simulink model "slexSysIdentMATLABSystemExample"  (R2017b)
settings: Solver=FixedStepDiscrete  StartTime=0.0  StopTime=1000  FixedStep=1  RelTol=1e-3
PreLoadFcn:
  | b = [ -0.0012   -0.0014    0.0020    0.0029   -0.0044   -0.0064    0.0090    0.0125 -0.0169   -0.0227    0.0305    0.0412   -0.0573   -0.0850    0.1472    0.4501 0.4501    0.1472   -0.0850   -0.0573    0.0412    0.0305   -0.0227   -0.0169 0.0125    0.0090   -0.0064   -0.0044    0.0029    0.0020   -0.0014   -0.0012];
  | N = 1;
InitFcn:
  | a = [zeros(1, N), b]; % Co-efficients of combined System (Unknown + Delay)
CloseFcn:
  | clear a b N
Description:
  | System Identification for an FIR System Using MATLAB System Blocks
  | 
  | This example shows how to use the MATLAB System block to implement
  | Simulink(R) blocks using a System object(TM). It highlights two MATLAB System blocks.
  | Access the MATLAB source code for each System object by clicking the "Source Code"
  | hyperlink from the block dialog.
  | 
  | * The Delay block uses a System object that has direct feedthrough
  | set to false. This implies that the System object does not directly use the input to
  | compute the output. Therefore, the Delay block could be safely used in a feedback system
  | without introducing an algebraic loop.
  | 
  | * The LMS Adaptive Filter block estimates the coefficients of an unknown system (formed
  | by the Unknown System and Delay blocks). Its inputs are the desired signal and
  | the actual signal. Its outputs are the estimated signal and the vector norm of the
  | error in the estimated coefficients.
  | 
  | * The Scope displays the error in the estimated signal and the vector norm
  | of the error in the estimated coefficients.
settings Model: ExtModeAutoUpdateStatusClock=off  Creator=The MathWorks, Inc.  LastModifiedBy=prave
settings DataIOCC: SaveFormat=Structure  SaveState=on
settings OptimizationCC: ExpressionDepthLimit=2147483647  InitFltsAndDblsToZero=on  LifeSpan=1
settings DebuggingCC: SaveWithParameterizedLinksMsg=none  UnderspecifiedInitializationDetection=Classic  MergeDetectMultiDrivingBlocksExec=none  SignalResolutionControl=TryResolveAllWithWarning  SolverPrmCheckMsg=warning  MultiTaskDSMMsg=warning  MultiTaskCondExecSysMsg=none  FcnCallInpInsideContextMsg=warning  AllowSymbolicDim=off  StateNameClashWarn=warning  SFUnexpectedBacktrackingDiag=warning  SFNoUnconditionalDefaultTransitionDiag=warning  SFExecutionAtInitializationDiag=none
settings HardwareCC: ProdBitPerPointer=32  ProdBitPerSizeT=32  ProdBitPerPtrDiffT=32  ProdLargestAtomicFloat=None  ProdIntDivRoundTo=Undefined  ProdEndianess=Unspecified  ProdWordSize=32  ProdHWDeviceType=32-bit Generic
settings ModelReferenceCC: PropagateSignalLabelsOutOfModel=off
settings SFSimCC: MATLABDynamicMemAlloc=off
settings RTWCC: SystemTargetFile=ert.tlc  TemplateMakefile=ert_default_tmf
settings CodeAppCC: IgnoreCustomStorageClasses=off  CustomSymbolStrType=$N$R$M  StateflowObjectComments=on  InternalIdentifier=Classic
settings ERTTargetCC: MultiwordLength=2048  GenerateSampleERTMain=on  ERTCustomFileTemplate=example_file_process.tlc  ConvertIfToSwitch=off  SuppressUnreachableDefaultCases=off
settings ConfigComp: CovMetricSettings=dw  CovHtmlReporting=on  CovSaveCumulativeToWorkspaceVar=on  CovSaveSingleToWorkspaceVar=on  CovExternalEMLEnable=off  CovSFcnEnable=off

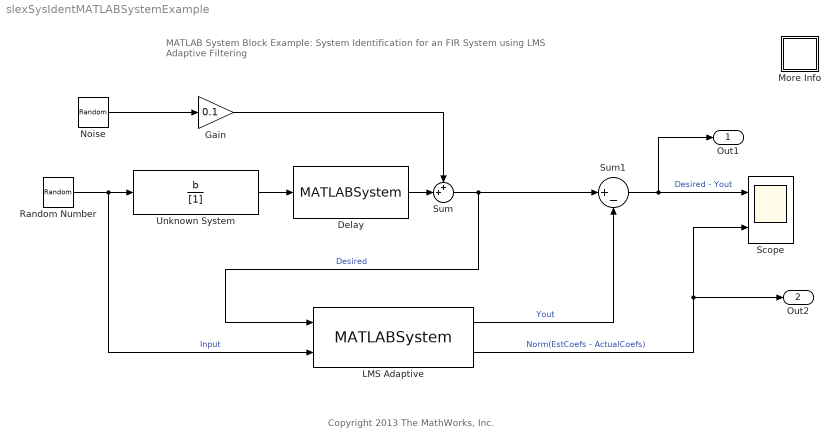
== system slexSysIdentMATLABSystemExample ==
  note: MATLAB System Block Example:
      | System Identification for an FIR System using LMS Adaptive Filtering
  note: Copyright 2013 The MathWorks, Inc.
  Delay : MATLABSystem  System=slexSysIdentMATLABSystemIntegerDelaySysObj  InitialOutput=0  NumberOfDelays=N  SimulateUsing=Code generation
      mask Type: slexSysIdentMATLABSystemIntegerDelaySysObj
      mask Display:
      | disp(['Integer' char(10) 'Delay']);
      | port_label('input',1,'inputs');
      | port_label('output',1,'outputs');
  Gain : Gain  Gain=0.1
  LMS Adaptive : MATLABSystem  System=slexSysIdentMATLABSystemLMSAdaptSysObj  Mu=0.005  SimulateUsing=Code generation  TrueCoefficients=a  NumCoefficients=numel(a)
      mask Type: slexSysIdentMATLABSystemLMSAdaptSysObj
      mask Display:
      | disp(['LMS Adaptive' char(10) 'Filter']);
      | port_label('input',1,'Desired');
      | port_label('input',2,'Actual');
      | port_label('output',1,'Output');
      | port_label('output',2,'EstError');
  More Info : Subsystem
      settings: OpenFcn=showdemo(bdroot(gcb))
      mask Display: disp('?')
  Noise : RandomNumber  Seed=3  SampleTime=1
  Random Number : RandomNumber  SampleTime=1
  Scope : Scope  NumInputPorts=2
  Sum : Sum  Inputs=++|
  Sum1 : Sum  Inputs=|+-
  Unknown System : DiscreteFilter  Numerator=b  Denominator=[1]
  Out1 : Outport
  Out2 : Outport  Port=2
  wires:
  Random Number/1 -> LMS Adaptive/2, Unknown System/1  "Input"
  Sum/1 -> LMS Adaptive/1, Sum1/1  "Desired"
  Sum1/1 -> Scope/1, Out1/1  "Desired - Yout"
  LMS Adaptive/1 -> Sum1/2  "Yout"
  LMS Adaptive/2 -> Scope/2, Out2/1  "Norm(EstCoefs - ActualCoefs)"
  Gain/1 -> Sum/1
  Noise/1 -> Gain/1
  Unknown System/1 -> Delay/1
  Delay/1 -> Sum/2

== system slexSysIdentMATLABSystemExample/More Info ==
  note: Bus Block Demonstration
  note: This demonstration shows how signals may be grouped and ungrouped while
      | retaining their names.  In this demonstration, 5 signals are created and labelled
      | appropriately.  These signals are then mux'd together to create a bus of signals.
      | This bus of signals is then fed into the Bus Selector block.  Inside of the Bus
      | Selector block, the Pulse and Chirp signals are chosen to be output from the
      | original signal bus.
      |
      | It is possible to place a nest signal buses and then still retrieve the original signal
      | with its label.
